simulink model "batteryCell"  (R2019a)
settings: Solver=VariableStepAuto  StartTime=0.0  StopTime=10.0  RelTol=1e-3
InitFcn:
  | load('batteryModelNew.mat');
  | load('soc_ocv_new.mat');
  | load('currentUAV.mat');
  | 
  | Q      = battery.QParam; % total capacity in mAh
  | n       = battery.etaParam; % coulombic efficiency
  | M      = battery.MParam; % dynamic hysteresis volts factor
  | Mo     = battery.M0Param; % instant hysteresis volts factor
  | Ro     = battery.R0Param; % internal resistance
  | R       = [battery.RCParam(1)]; % diffusion / warburg impedence, pairs with C
  | C       = [battery.RCParam(2)]; % diffusion / warburg impedence, pairs with R
  | g       = battery.GParam;  % gamma, tunes decay in hysteresis
  | dt      = .01; % delta t
  | eod   = battery.EODParam; % final voltage
  | 
  | if length(R) ~= length(C)
  |     error("R and C must be the same length");
  | end
  | 
  | Arc = zeros(length(R));
  | for i = 1:length(R)
  |     Arc(i,i) = exp(-dt/(R(i)*C(i)));
  | end
  | Brc = zeros(length(R), 1);
  | for i = 1:length(R)
  |     Brc(i,1) = 1 - exp(-dt/(R(i)*C(i)));
  | end
  | k = 1; % timestep
  | Io = .1; % current at time k
  | H(k) = exp(-abs((n(k)*Io(k)*g*dt)/Q));
  | 
  | 
  | %Io = current(1:floor(length(current)/2.5));
  | Io = current;
  | %Io = 0.0;
  | 
  | z = 1.0; % soc
  | Ir = zeros(length(R), 1);
  | h = 0.0;
  | v = ones(length(Io));
  | 
  | 
  | soc = zeros(1, length(Io));
  | v = soc;
values from neighbouring files (symbols this model uses):
  battery =     [batteryModel.mat]
  soc_ocv = [3.01299571991 3.22696254321 3.33372423053 3.41002026482 3.47185878204 3.52366305014 3.56834682613 3.60755277958 3.64212119234 3.67146891607 3.6938685759 3.70622742565 ... (101 elements, 1x101)]    [soc_ocv.mat]
settings Model: Creator=tdarrah  LastModifiedBy=tdarrah

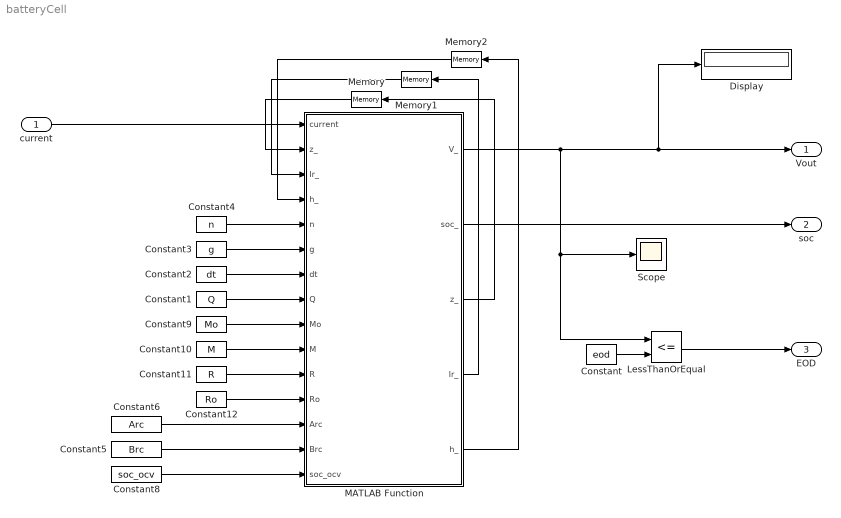
== system batteryCell ==
  current : Inport
  Constant : Constant  Value=eod
  Constant1 : Constant  Value=Q
  Constant10 : Constant  Value=M
  Constant11 : Constant  Value=R
  Constant12 : Constant  Value=Ro
  Constant2 : Constant  Value=dt
  Constant3 : Constant  Value=g
  Constant4 : Constant  Value=n
  Constant5 : Constant  Value=Brc
  Constant6 : Constant  Value=Arc
  Constant8 : Constant  Value=soc_ocv
  Constant9 : Constant  Value=Mo
  Display : Display
  LessThanOrEqual : RelationalOperator  Operator=<=  OutDataTypeStr=boolean  RndMeth=Simplest
  MATLAB Function : MATLAB Function  TreatAsAtomicUnit=on
  Memory : Memory  InitialCondition=1
  Memory1 : Memory
  Memory2 : Memory
  Scope : Scope
  Vout : Outport
  soc : Outport  Port=2
  EOD : Outport  Port=3
  wires:
  Constant6/1 -> MATLAB Function/13(Arc)
  Memory1/1 -> MATLAB Function/3("Ir_ ")
  Constant9/1 -> MATLAB Function/9(Mo)
  Constant10/1 -> MATLAB Function/10(M)
  MATLAB Function/1(V_) -> Scope/1, LessThanOrEqual/1, Display/1, Vout/1
  current/1 -> MATLAB Function/1(current)
  MATLAB Function/4(Ir_) -> Memory1/1
  Constant12/1 -> MATLAB Function/12(Ro)
  Constant11/1 -> MATLAB Function/11(R)
  Constant3/1 -> MATLAB Function/6(g)
  Constant1/1 -> MATLAB Function/8(Q)
  MATLAB Function/3(z_) -> Memory/1
  Memory2/1 -> MATLAB Function/4("h_ ")
  MATLAB Function/2(soc_) -> soc/1
  Constant5/1 -> MATLAB Function/14(Brc)
  MATLAB Function/5(h_) -> Memory2/1
  Memory/1 -> MATLAB Function/2("z_ ")
  Constant2/1 -> MATLAB Function/7(dt)
  Constant/1 -> LessThanOrEqual/2
  Constant8/1 -> MATLAB Function/15(soc_ocv)
  LessThanOrEqual/1 -> EOD/1
  Constant4/1 -> MATLAB Function/5(n)

== matlab function batteryCell/MATLAB Function ==
  data: current input; V_ output; z_ input; Ir_ input; h_ input; soc_ output; z_ output; Ir_ output; h_ output; n input; g input; dt input; Q input; Mo input; M input; R input; Ro input; Arc input; Brc input; soc_ocv input
function [V_, soc_, z_, Ir_, h_]= batterySim(current, z_, Ir_, h_, n, g, dt, Q, Mo, M, R, Ro, Arc, Brc, soc_ocv)
    soc_ = 1.0;
    V_ = 4.2;
    z_dot = z_ - ((n*dt)/Q)*current;
    Ir_dot = Arc*Ir_ + Brc*current;
    H = exp(-abs((n*current*g*dt)/Q));
    h_dot = H*h_ + (H-1)*sign(current);
    z_ = z_dot;
    Ir_ = Ir_dot;
    h_ = h_dot;
    soc_ = (z_ + 31.8816) /(1.0 + 31.8816);
    idx = ceil(soc_*100) +1;
    V_ = (soc_ocv(idx) + Mo*sign(current) + M*h_ - sum(R*Ir_) - Ro*current);
